simulink model "C172S_AutopilotModeManager_V1"  (R2026a)
settings: Solver=FixedStepDiscrete  StartTime=0  StopTime=3  FixedStep=0.01
InitFcn:
  | amm1Manager = c172sAutopilotModeManagerData();
  | if ~strcmp(amm1Manager.artifactRevision,'AUTOPILOT-MODE-MANAGER-V1-AUDIT-MATLAB-R1'), error('Mode Manager V1 artifact mismatch.'); end
  | if ~exist('amm1InputSignal','var'), error('amm1InputSignal is required.'); end
settings Model: Creator=Shahi  LastModifiedBy=Shahi

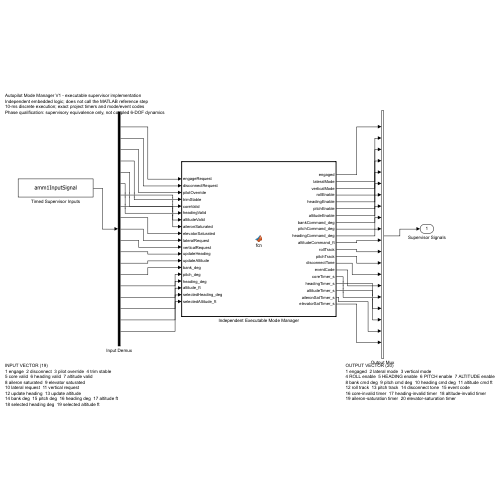
[thumbnail: Simulink's stored preview of the top-level diagram]
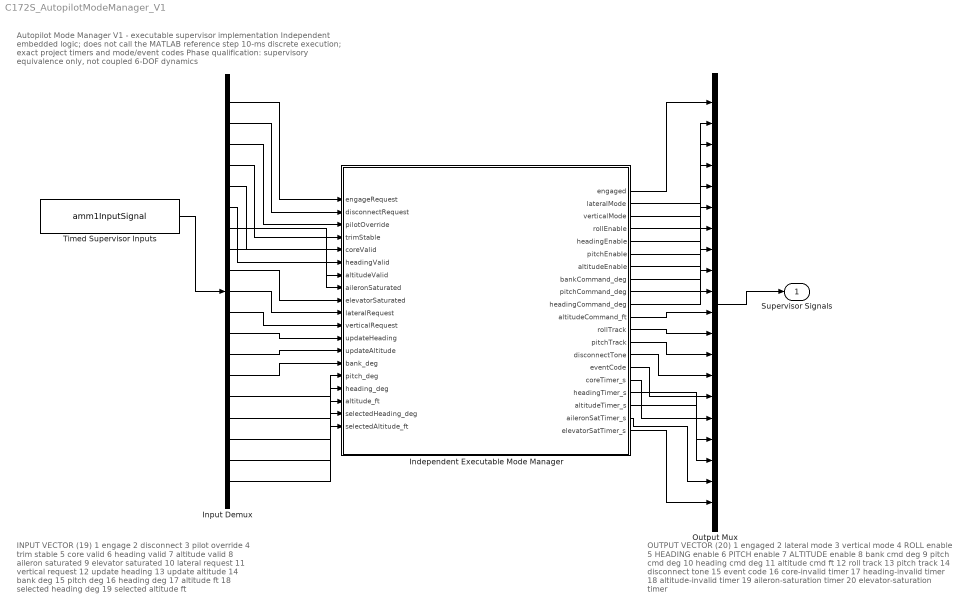
== system C172S_AutopilotModeManager_V1 ==
  note: Autopilot Mode Manager V1 - executable supervisor implementation
      | Independent embedded logic; does not call the MATLAB reference step
      | 10-ms discrete execution; exact project timers and mode/event codes
      | Phase qualification: supervisory equivalence only, not coupled 6-DOF dynamics
  note: INPUT VECTOR (19)
      | 1 engage  2 disconnect  3 pilot override  4 trim stable
      | 5 core valid  6 heading valid  7 altitude valid
      | 8 aileron saturated  9 elevator saturated
      | 10 lateral request  11 vertical request
      | 12 update heading  13 update altitude
      | 14 bank deg  15 pitch deg  16 heading deg  17 altitude ft
      | 18 selected heading deg  19 selected altitude ft
  note: OUTPUT VECTOR (20)
      | 1 engaged  2 lateral mode  3 vertical mode
      | 4 ROLL enable  5 HEADING enable  6 PITCH enable  7 ALTITUDE enable
      | 8 bank cmd deg  9 pitch cmd deg  10 heading cmd deg  11 altitude cmd ft
      | 12 roll track  13 pitch track  14 disconnect tone  15 event code
      | 16 core-invalid timer  17 heading-invalid timer  18 altitude-invalid timer
      | 19 aileron-saturation timer  20 elevator-saturation timer
  Independent Executable Mode Manager : MATLAB Function  TreatAsAtomicUnit=on
  Input Demux : Demux  Outputs=19
  Output Mux : Mux  Inputs=20
  Timed Supervisor Inputs : FromWorkspace  VariableName=amm1InputSignal  SampleTime=0.01  Interpolate=off  OutputAfterFinalValue=Holding final value
  Supervisor Signals : Outport
  wires:
  Input Demux/1 -> Independent Executable Mode Manager/1(engageRequest)
  Input Demux/2 -> Independent Executable Mode Manager/2(disconnectRequest)
  Input Demux/3 -> Independent Executable Mode Manager/3(pilotOverride)
  Input Demux/4 -> Independent Executable Mode Manager/4(trimStable)
  Input Demux/5 -> Independent Executable Mode Manager/5(coreValid)
  Input Demux/6 -> Independent Executable Mode Manager/6(headingValid)
  Input Demux/7 -> Independent Executable Mode Manager/7(altitudeValid)
  Input Demux/8 -> Independent Executable Mode Manager/8(aileronSaturated)
  Input Demux/9 -> Independent Executable Mode Manager/9(elevatorSaturated)
  Input Demux/10 -> Independent Executable Mode Manager/10(lateralRequest)
  Input Demux/11 -> Independent Executable Mode Manager/11(verticalRequest)
  Input Demux/12 -> Independent Executable Mode Manager/12(updateHeading)
  Input Demux/13 -> Independent Executable Mode Manager/13(updateAltitude)
  Input Demux/14 -> Independent Executable Mode Manager/14(bank_deg)
  Input Demux/15 -> Independent Executable Mode Manager/15(pitch_deg)
  Input Demux/16 -> Independent Executable Mode Manager/16(heading_deg)
  Input Demux/17 -> Independent Executable Mode Manager/17(altitude_ft)
  Input Demux/18 -> Independent Executable Mode Manager/18(selectedHeading_deg)
  Input Demux/19 -> Independent Executable Mode Manager/19(selectedAltitude_ft)
  Independent Executable Mode Manager/1(engaged) -> Output Mux/1
  Independent Executable Mode Manager/2(lateralMode) -> Output Mux/2
  Independent Executable Mode Manager/3(verticalMode) -> Output Mux/3
  Independent Executable Mode Manager/4(rollEnable) -> Output Mux/4
  Independent Executable Mode Manager/5(headingEnable) -> Output Mux/5
  Independent Executable Mode Manager/6(pitchEnable) -> Output Mux/6
  Independent Executable Mode Manager/7(altitudeEnable) -> Output Mux/7
  Independent Executable Mode Manager/8(bankCommand_deg) -> Output Mux/8
  Independent Executable Mode Manager/9(pitchCommand_deg) -> Output Mux/9
  Independent Executable Mode Manager/10(headingCommand_deg) -> Output Mux/10
  Independent Executable Mode Manager/11(altitudeCommand_ft) -> Output Mux/11
  Independent Executable Mode Manager/12(rollTrack) -> Output Mux/12
  Independent Executable Mode Manager/13(pitchTrack) -> Output Mux/13
  Independent Executable Mode Manager/14(disconnectTone) -> Output Mux/14
  Independent Executable Mode Manager/15(eventCode) -> Output Mux/15
  Independent Executable Mode Manager/16(coreTimer_s) -> Output Mux/16
  Independent Executable Mode Manager/17(headingTimer_s) -> Output Mux/17
  Independent Executable Mode Manager/18(altitudeTimer_s) -> Output Mux/18
  Independent Executable Mode Manager/19(aileronSatTimer_s) -> Output Mux/19
  Independent Executable Mode Manager/20(elevatorSatTimer_s) -> Output Mux/20
  Timed Supervisor Inputs/1 -> Input Demux/1
  Output Mux/1 -> Supervisor Signals/1

== matlab function C172S_AutopilotModeManager_V1/Independent Executable Mode Manager ==
  data: engageRequest input; engaged output; disconnectRequest input; pilotOverride input; trimStable input; coreValid input; headingValid input; altitudeValid input; aileronSaturated input; elevatorSaturated input; lateralRequest input; verticalRequest input; updateHeading input; updateAltitude input; bank_deg input; pitch_deg input; heading_deg input; altitude_ft input; selectedHeading_deg input; selectedAltitude_ft input; lateralMode output; verticalMode output; rollEnable output; headingEnable output; pitchEnable output; altitudeEnable output; bankCommand_deg output; pitchCommand_deg output; headingCommand_deg output; altitudeCommand_ft output; rollTrack output; pitchTrack output; disconnectTone output; eventCode output; coreTimer_s output; headingTimer_s output; altitudeTimer_s output; aileronSatTimer_s output; elevatorSatTimer_s output
function [engaged,lateralMode,verticalMode,rollEnable,headingEnable,pitchEnable,altitudeEnable,bankCommand_deg,pitchCommand_deg,headingCommand_deg,altitudeCommand_ft,rollTrack,pitchTrack,disconnectTone,eventCode,coreTimer_s,headingTimer_s,altitudeTimer_s,aileronSatTimer_s,elevatorSatTimer_s] = supervisor(engageRequest,disconnectRequest,pilotOverride,trimStable,coreValid,headingValid,altitudeValid,aileronSaturated,elevatorSaturated,lateralRequest,verticalRequest,updateHeading,updateAltitude,bank_deg,pitch_deg,heading_deg,altitude_ft,selectedHeading_deg,selectedAltitude_ft)
%#codegen
persistent ap lat vert bankRef pitchRef headingRef altitudeRef
persistent coreTimer headingTimer altitudeTimer aileronTimer elevatorTimer
if isempty(ap)
    ap = false; lat = 0; vert = 0;
    bankRef = captureBank(bank_deg); pitchRef = capturePitch(pitch_deg);
    headingRef = normalizeHeading(heading_deg); altitudeRef = altitude_ft;
    coreTimer = 0.0; headingTimer = 0.0; altitudeTimer = 0.0;
    aileronTimer = 0.0; elevatorTimer = 0.0;
end
dt = 0.01;
eventCode = 0; rollTrack = 0; pitchTrack = 0; disconnectTone = 0;
wasEngaged = ap;
coreTimer = timerUpdate(coreValid < 0.5,coreTimer,dt);
headingTimer = timerUpdate(headingValid < 0.5,headingTimer,dt);
altitudeTimer = timerUpdate(altitudeValid < 0.5,altitudeTimer,dt);
aileronTimer = timerUpdate(aileronSaturated > 0.5,aileronTimer,dt);
elevatorTimer = timerUpdate(elevatorSaturated > 0.5,elevatorTimer,dt);
if ap
    if disconnectRequest > 0.5
        ap = false; lat = 0; vert = 0; eventCode = 7; disconnectTone = 1;
    elseif pilotOverride > 0.5
        ap = false; lat = 0; vert = 0; eventCode = 8; disconnectTone = 1;
    elseif abs(bank_deg) > 30 || abs(pitch_deg) > 10
        ap = false; lat = 0; vert = 0; eventCode = 11; disconnectTone = 1;
    elseif coreTimer + 1.0e-12 >= 0.10000000000000001
        ap = false; lat = 0; vert = 0; eventCode = 9; disconnectTone = 1;
    elseif max(aileronTimer,elevatorTimer) + 1.0e-12 >= 2
        ap = false; lat = 0; vert = 0; eventCode = 10; disconnectTone = 1;
    end
end
if ~ap
    if ~wasEngaged && engageRequest > 0.5
        permitted = trimStable > 0.5 && coreValid > 0.5 && pilotOverride < 0.5 && aileronSaturated < 0.5 && elevatorSaturated < 0.5;
        if lateralRequest == 2, permitted = permitted && headingValid > 0.5; end
        if verticalRequest == 2, permitted = permitted && altitudeValid > 0.5; end
        if permitted
            ap = true; eventCode = 1; rollTrack = 1; pitchTrack = 1;
            if lateralRequest == 2
                lat = 2; headingRef = normalizeHeading(selectedHeading_deg);
            else
                lat = 1; bankRef = captureBank(bank_deg);
            end
            if verticalRequest == 2
                vert = 2; altitudeRef = selectedAltitude_ft;
            else
                vert = 1; pitchRef = capturePitch(pitch_deg);
            end
        else
            eventCode = 4;
        end
    end
else
    if lat == 2 && headingTimer + 1.0e-12 >= 0.10000000000000001
        lat = 1; bankRef = captureBank(bank_deg); rollTrack = 1; eventCode = 5;
    end
    if vert == 2 && altitudeTimer + 1.0e-12 >= 0.10000000000000001
        vert = 1; pitchRef = capturePitch(pitch_deg); pitchTrack = 1; eventCode = 6;
    end
    if lateralRequest ~= 0
        if lateralRequest == 1
            lat = 1; bankRef = captureBank(bank_deg); rollTrack = 1; eventCode = 2;
        elseif lateralRequest == 2 && headingValid > 0.5
            lat = 2; headingRef = normalizeHeading(selectedHeading_deg); rollTrack = 1; eventCode = 2;
        else
            eventCode = 3;
        end
    end
    if verticalRequest ~= 0
        if verticalRequest == 1
            vert = 1; pitchRef = capturePitch(pitch_deg); pitchTrack = 1; eventCode = 2;
        elseif verticalRequest == 2 && altitudeValid > 0.5
            vert = 2; altitudeRef = selectedAltitude_ft; pitchTrack = 1; eventCode = 2;
        else
            eventCode = 3;
        end
    end
    if lat == 2 && updateHeading > 0.5 && headingValid > 0.5
        headingRef = normalizeHeading(selectedHeading_deg);
    end
    if vert == 2 && updateAltitude > 0.5 && altitudeValid > 0.5
        altitudeRef = selectedAltitude_ft;
    end
end
engaged = double(ap); lateralMode = lat; verticalMode = vert;
rollEnable = double(ap && lat == 1); headingEnable = double(ap && lat == 2);
pitchEnable = double(ap && vert == 1); altitudeEnable = double(ap && vert == 2);
bankCommand_deg = 0.0; pitchCommand_deg = 0.0;
if ap && lat == 1, bankCommand_deg = bankRef; end
if ap && vert == 1, pitchCommand_deg = pitchRef; end
headingCommand_deg = headingRef; altitudeCommand_ft = altitudeRef;
coreTimer_s = coreTimer; headingTimer_s = headingTimer; altitudeTimer_s = altitudeTimer;
aileronSatTimer_s = aileronTimer; elevatorSatTimer_s = elevatorTimer;
end
function value = captureBank(value)
if abs(value) < 6
    value = 0.0;
else
    value = min(max(value,-20),20);
end
end
function value = capturePitch(value)
value = min(max(value,-3),3);
end
function value = normalizeHeading(value)
value = mod(value,360.0);
if value < 0.0, value = value + 360.0; end
end
function timer = timerUpdate(condition,timer,dt)
if condition, timer = timer + dt; else, timer = 0.0; end
end
